simulink model "FogRectificationHDL"  (R2024b)
settings: Solver=FixedStepDiscrete  StartTime=0.0  StopTime=2*T  RelTol=1e-3
InitFcn:
  | img_path = get_param('FogRectificationHDL/FogImage','FileName');
  | img = imread(img_path);
  | %[m,n,c] = size(img);
  | m = 240;
  | n = 320;
  | c = 3;
  | dimI = [m n 3];
  | g = m*n;
  | 
  | numPixels = prod(dimI);
  | h1 = [1, 2, 1; 2, 4, 2; 1, 2 ,1]./16 ;
  | h = fliplr(flipud(h1));
  | T =324*402; % total pixels per line*total video lines
  | 
  | numBins = 256;
  | hazeFactor = 0.9;
  | reductionFactor = 0.6;
  | normFactor =  1/g;
  | threshold1 = 0.05;
  | threshold2 = 0.95;
  | o1 = 25;
  | o2 = 229;
  | o2_1 = 204;
  | max_o2 = 26;
undefined symbols (not defined in the file or in its folder): gray, Rec, SDTV
libraries: simulink x40, hdlsllib x32, visionhdlutilities x2, visionhdlio x2, visionsources x1, visionhdlstatistics x1, visionhdlconversions x1, visionhdlfilter x1, visionzynq_privlib x1
(part 1 of 2)
settings Model: DataTypeOverride=Off  ModifiedByFormat=The MathWorks, Inc.  SimulationMode=accelerator  Creator=The MathWorks, Inc.  LastModifiedBy=The MathWorks, Inc.
settings SolverCC: AlgebraicLoopSolver=TrustRegion
settings DataIOCC: SaveOutput=off  SaveTime=off
settings OptimizationCC: BlockReduction=off  ConditionallyExecuteInputs=off  DefaultParameterBehavior=Inlined
settings DebuggingCC: AlgebraicLoopMsg=error  SingleTaskRateTransMsg=error  ParameterPrecisionLossMsg=none  UnconnectedInputMsg=warning  UnconnectedOutputMsg=warning  UnconnectedLineMsg=warning
settings HardwareCC: ProdBitPerPointer=32  ProdBitPerSizeT=32  ProdBitPerPtrDiffT=32  ProdLargestAtomicFloat=None  ProdIntDivRoundTo=Undefined  ProdEndianess=Unspecified  ProdWordSize=32  ProdHWDeviceType=ASIC/FPGA->ASIC/FPGA  TargetBitPerLong=64  TargetBitPerPointer=64  TargetBitPerSizeT=64  TargetBitPerPtrDiffT=64  TargetLongLongMode=on  TargetIntDivRoundTo=Zero  TargetEndianess=LittleEndian  TargetWordSize=64  TargetHWDeviceType=Custom Processor->MATLAB Host Computer  ProdEqTarget=off
settings ModelReferenceCC: EnableRefExpFcnMdlSchedulingChecks=on
settings RTWCC: GPUComputeCapability=3.5  DLArmComputeVersion=19.05

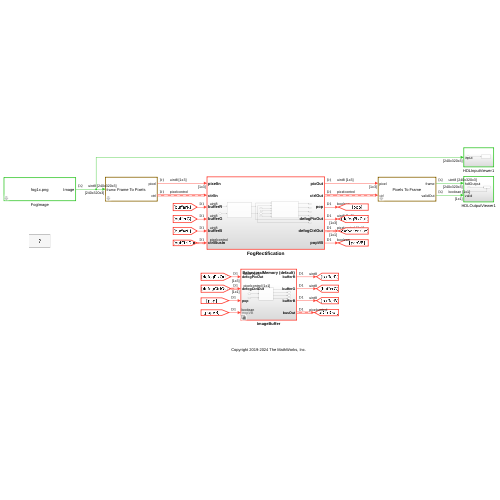
[thumbnail: Simulink's stored preview of the top-level diagram]
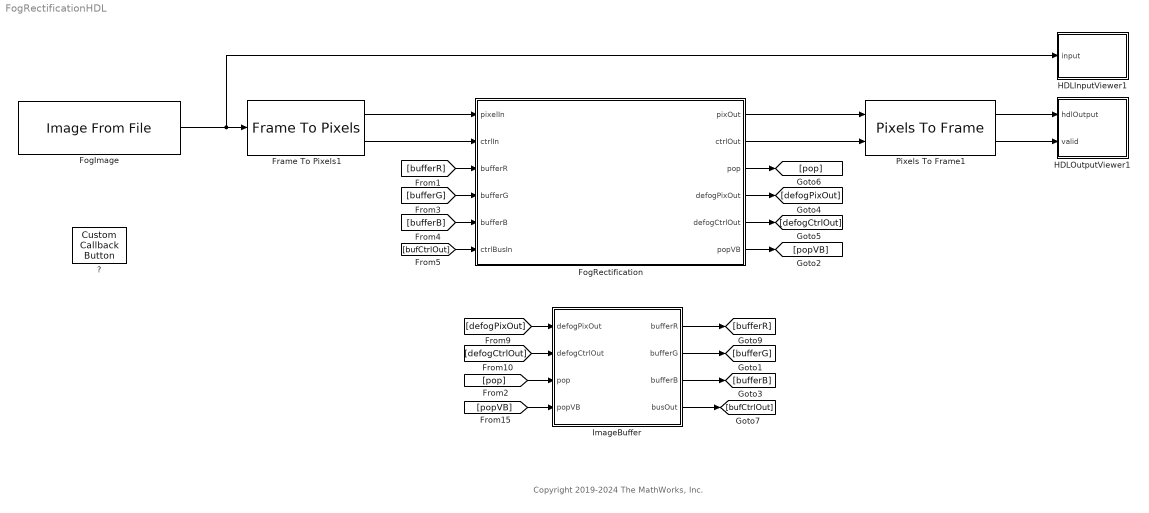
== system FogRectificationHDL ==
  note: Copyright 2019-2024 The MathWorks, Inc.
  "?" : CustomCallbackButton  Configuration="{\"components\":[{\"name\":\"BackgroundImageComponent\",\"settings\":{\"image\":{\"size\":[0,0],\"src\":\"default\",\"srcOrientation\":\"Right\"},\"position\":[0,0,1,1]}},{\"name\":\"ButtonStateComponent\",\"settings\":{\"buttonType\":\"momentary\",\"clickFcn\":\"showExample('visionhdl\\/FogRectificationHDLExample')\",\"onValue\":1,\"position\":[0,0,1,1],\"pressDelay\":\"500\",\"pressFcn\":\"\",\"repeatInterval\":\"0\",\"states\":[{\"horizontalAlignment\":\"center\",\"image\":{\"position\":[0,0,1,1],\"size\":[1,1],\"src\":\"default\",\"srcOrientation\":\"Right\"},\"label\":{\"color\":[0.01176470588,0.01176470588,0.01176470588,1],\"icon\":{\"size\":[0,0],\"src\":\"default\",\"srcOrientation\":\"Right\"},\"iconPlacement\":\"left\",\"opacity\":1,\"show\":true,\"text\":{\"content\":\"?\",\"font\":\"Helvetica\"}},\"labelOffset\":[0,0],\"verticalAlignment\":\"middle\"},{\"horizontalAlignment\":\"center\",\"image\":{\"position\":[0,0,1,1],\"size\":[1,1],\"src\":\"default\",\"srcOrientation\":\"Right\"},\"label\":{\"color\":[0.01176470588,0.01176470588,0.01176470588,1],\"icon\":{\"size\":[0,0],\"src\":\"default\",\"srcOrientation\":\"Right\"},\"iconPlacement\":\"left\",\"opacity\":1,\"show\":true,\"text\":{\"content\":\"?\",\"font\":\"Helvetica\"}},\"labelOffset\":[0,0],\"verticalAlignment\":\"middle\"},{\"horizontalAlignment\":\"center\",\"image\":{\"position\":[0,0,1,1],\"size\":[1,1],\"src\":\"default\",\"srcOrientation\":\"Right\"},\"label\":{\"color\":[0.01176470588,0.01176470588,0.01176470588,1],\"icon\":{\"size\":[0,0],\"src\":\"default\",\"srcOrientation\":\"Right\"},\"iconPlacement\":\"left\",\"opacity\":1,\"show\":true,\"text\":{\"content\":\"?\",\"font\":\"Helvetica\"}},\"labelOffset\":[0,0],\"verticalAlignment\":\"middle\"},{\"horizontalAlignment\":\"center\",\"image\":{\"position\":[0,0,1,1],\"size\":[1,1],\"src\":\"default\",\"srcOrientation\":\"Right\"},\"label\":{\"color\":[0.01176470588,0.01176470588,0.01176470588,1],\"icon\":{\"size\":[0,0],\"src\":\"default\",\"srcOrientation\":\"Right\"},\"iconPlacement\":\"left\",\"opacity\":1,\"show\":true,\"text\":{\"content\":\"?\",\"font\":\"Helvetica\"}},\"labelOffset\":[0,0],\"verticalAlignment\":\"middle\"}]}},{\"name\":\"ForegroundImageComponent\",\"settings\":{\"image\":{\"size\":[0,0],\"src\":\"default\",\"srcOrientation\":\"Right\"},\"isForeground\":1,\"position\":[0,0,1,1]}}],\"settings\":{\"BindingType\":\"standalone\",\"backgroundColor\":[244,244,244,1],\"backgroundOffset\":0,\"backgroundOpacity\":1,\"fixedAspectRatio\":\"off\",\"foregroundColor\":[0.01176470588,0.01176470588,0.01176470588,1],\"migratedFromLegacy\":true,\"useBackgroundColor\":true,\"variant\":\"callback\",\"version\":\"R2024b\"},\"type\":\"Button\"}"  CustomBackgroundColor="{\"color\":[0.9568627451,0.9568627451,0.9568627451],\"show\":true}"
  FogImage : visionsources/Image From File  Tag=vipblks_nd  FileName=./fog1x.png  Ts=T  imagePorts=One multidimensional signal  OutPortLabels=R|G|B  ImageDataType=Inherit from input image  sdImageDataType=uint(8)  Signed=on  WordLength=16  FractionLengthMode=User-defined  FractionLength=15
  FogRectification : Subsystem
  Frame To Pixels1 : visionhdlio/Frame To Pixels  NumComponents=3  NumPixels=1  VideoFormat=240p  ActivePixelsPerLine=320  ActiveVideoLines=240  TotalPixelsPerLine=402  TotalVideoLines=324  StartingActiveLine=1  FrontPorch=44  SampleTime=0  VideoFormatCache=240p  ActivePixelsPerLineCache=160  ActiveVideoLinesCache=160  TotalPixelsPerLineCache=400  TotalVideoLinesCache=400  StartingActiveLineCache=6  FrontPorchCache=120
  HDLInputViewer1 : Subsystem
  HDLOutputViewer1 : Subsystem
  ImageBuffer : Subsystem  Variant=on  VariantControlMode=label  LabelModeActiveChoice=(default)
  Pixels To Frame1 : visionhdlio/Pixels To Frame  NumComponents=3  NumPixels=1  VideoFormat=240p  ActivePixelsPerLine=320  ActiveVideoLines=240  TotalPixelsPerLine=402  TotalVideoLines=324  VideoFormatCache=240p  ActivePixelsPerLineCache=320  ActiveVideoLinesCache=240  TotalPixelsPerLineCache=402  TotalVideoLinesCache=324
  wires:
  FogRectification/6(popVB) -> [popVB]
  FogRectification/1(pixOut) -> Pixels To Frame1/1
  FogImage/1 -> HDLInputViewer1/1(input), Frame To Pixels1/1
  Pixels To Frame1/2 -> HDLOutputViewer1/2(valid)
  FogRectification/3(pop) -> [pop]
  [bufferR] -> FogRectification/3(bufferR)
  FogRectification/2(ctrlOut) -> Pixels To Frame1/2
  Pixels To Frame1/1 -> HDLOutputViewer1/1(hdlOutput)
  ImageBuffer/3(bufferB) -> [bufferB]
  [pop] -> ImageBuffer/3(pop)
  Frame To Pixels1/1 -> FogRectification/1(pixelIn)
  ImageBuffer/2(bufferG) -> [bufferG]
  Frame To Pixels1/2 -> FogRectification/2(ctrlIn)
  [bufferB] -> FogRectification/5(bufferB)
  FogRectification/5(defogCtrlOut) -> [defogCtrlOut]
  [defogPixOut] -> ImageBuffer/1(defogPixOut)
  FogRectification/4(defogPixOut) -> [defogPixOut]
  ImageBuffer/4(busOut) -> [bufCtrlOut]
  [popVB] -> ImageBuffer/4(popVB)
  ImageBuffer/1(bufferR) -> [bufferR]
  [defogCtrlOut] -> ImageBuffer/2(defogCtrlOut)
  [bufCtrlOut] -> FogRectification/6(ctrlBusIn)
  [bufferG] -> FogRectification/4(bufferG)

== system FogRectificationHDL/FogRectification ==
  pixelIn : Inport
  ctrlIn : Inport  Port=2
  bufferR : Inport  Port=3
  bufferG : Inport  Port=4
  bufferB : Inport  Port=5
  ctrlBusIn : Inport  Port=6
  ContrastEnhancement : Subsystem
  FogRemoval : Subsystem
  pixOut : Outport  VectorParamsAs1DForOutWhenUnconnected=off
  ctrlOut : Outport  Port=2  VectorParamsAs1DForOutWhenUnconnected=off
  pop : Outport  Port=3  VectorParamsAs1DForOutWhenUnconnected=off
  defogPixOut : Outport  Port=4  VectorParamsAs1DForOutWhenUnconnected=off
  defogCtrlOut : Outport  Port=5  VectorParamsAs1DForOutWhenUnconnected=off
  popVB : Outport  Port=6  VectorParamsAs1DForOutWhenUnconnected=off
  wires:
  pixelIn/1 -> FogRemoval/1(pixelIn)
  ctrlIn/1 -> FogRemoval/2(ctrlIn)
  FogRemoval/1(defogPixOut) -> ContrastEnhancement/1(pixelIn), defogPixOut/1
  FogRemoval/2(defogCtrlOut) -> ContrastEnhancement/2(ctrlIn), defogCtrlOut/1
  bufferR/1 -> ContrastEnhancement/3(bufferR)
  bufferG/1 -> ContrastEnhancement/4(bufferG)
  bufferB/1 -> ContrastEnhancement/5(bufferB)
  ContrastEnhancement/1(pixelOut) -> pixOut/1
  ContrastEnhancement/2(ctrlBusOut) -> ctrlOut/1
  ContrastEnhancement/3(pop) -> pop/1
  ctrlBusIn/1 -> ContrastEnhancement/6(ctrlBusIn)
  ContrastEnhancement/4(popVB) -> popVB/1

== system FogRectificationHDL/HDLInputViewer1 ==
  input : Inport
  hdlFogInput : VideoViewer  colormapValue=gray(256)  FigPos=[1217 942 673 613]
  wires:
  input/1 -> hdlFogInput/1

== system FogRectificationHDL/HDLOutputViewer1 ==
  hdlOutput : Inport
  valid : Inport  Port=2
  HDLOutputViewer : Subsystem
  wires:
  hdlOutput/1 -> HDLOutputViewer/1(h)
  valid/1 -> HDLOutputViewer/Enable

== system FogRectificationHDL/ImageBuffer ==
  note: 1) Add Subsystem or Model blocks as valid variant choices.
      | 2) You cannot connect blocks at this level. At simulation, connectivity is automatically
      | determined, based on the active variant and port name matching.
  note: 1) Behavioral Memory and VideoFrameBuffer are the two variant choices.
      | 2) Behavioral Memory is designed using HDL FIFO blocks.
      | 3) VideoFrameBuffer block is used from xilinxzynqbasedvision supportPkg.
      | 4) Currently VideoFrameBuffer block is used only for Simulation.
      | 5) For FPGA-in-the-Loop Simulations, make sure Behavioral Memory is enabled.
  defogPixOut : Inport
  defogCtrlOut : Inport  Port=2
  pop : Inport  Port=3
  popVB : Inport  Port=4
  BehavioralMemory : Subsystem  VariantControl=(default)
  VideoFrameBuffer : Subsystem  VariantControl=VideoFrameBuffer
  bufferR : Outport
  bufferG : Outport  Port=2
  bufferB : Outport  Port=3
  busOut : Outport  Port=4

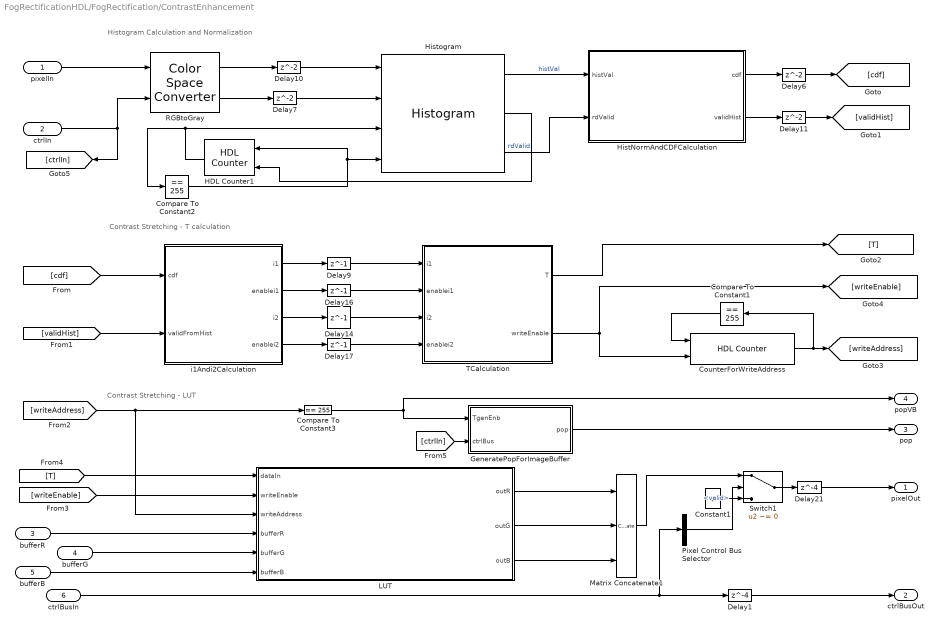
== system FogRectificationHDL/FogRectification/ContrastEnhancement ==
  note: Histogram Calculation and Normalization
  note: Contrast Stretching - LUT
  note: Contrast Stretching - T calculation
  pixelIn : Inport
  ctrlIn : Inport  Port=2
  bufferR : Inport  Port=3
  bufferG : Inport  Port=4
  bufferB : Inport  Port=5
  ctrlBusIn : Inport  Port=6
  Compare To Constant1 : simulink/Logic and Bit Operations/Compare To Constant  relop===  const=255  OutDataTypeStr=boolean
  Compare To Constant2 : simulink/Logic and Bit Operations/Compare To Constant  relop===  const=255  OutDataTypeStr=boolean
  Compare To Constant3 : simulink/Logic and Bit Operations/Compare To Constant  relop===  const=255  OutDataTypeStr=boolean
  Constant1 : Constant  Value=0  OutDataTypeStr=uint8  SampleTime=-1
  CounterForWriteAddress : hdlsllib/Sources/HDL Counter  CountType=Free running  CountInit=0  CountStep=1  CountMax=25  CountFromType=Initial value  CountFrom=0  CountResetPort=on  CountLoadPort=off  CountEnbPort=on  CountDirPort=off  CountHitOutputPort=off  CountDataType=Unsigned  CountWordLen=8  CountFracLen=0  CountSampTime=1
  Delay1 : Delay  DelayLength=4
  Delay{6..7,10..11} (4 alike) : Delay
  Delay{9,14,16..17} (4 alike) : Delay  DelayLength=1
  Delay21 : Delay  DelayLength=4
  GeneratePopForImageBuffer : Subsystem
  HDL Counter1 : hdlsllib/Sources/HDL Counter  CountType=Count limited  CountInit=0  CountStep=1  CountMax=255  CountFromType=Initial value  CountFrom=0  CountResetPort=on  CountLoadPort=off  CountEnbPort=on  CountDirPort=off  CountHitOutputPort=off  CountDataType=Unsigned  CountWordLen=ceil(log2(numBins))  CountFracLen=0  CountSampTime=1
  HistNormAndCDFCalculation : Subsystem
  Histogram : visionhdlstatistics/Histogram  NumBins=256  OutputDataType=Unsigned fixed point  OutputWL=16  SimulateUsing=Code generation
  LUT : Subsystem
  Matrix Concatenate1 : Concatenate  NumInputs=3  Mode=Multidimensional array  ConcatenateDimension=2
  Pixel Control Bus Selector : BusSelector  OutputSignals=valid
  RGBtoGray : visionhdlconversions/Color Space Converter  Conversion=RGB to intensity  ConversionStandard=Rec. 601 (SDTV)  ScanningStandard=1250/50/2:1  SimulateUsing=Code generation
  Switch1 : Switch  Criteria=u2 ~= 0  SaturateOnIntegerOverflow=off  InputSameDT=off
  TCalculation : Subsystem
  i1Andi2Calculation : Subsystem
  pixelOut : Outport
  ctrlBusOut : Outport  Port=2
  pop : Outport  Port=3
  popVB : Outport  Port=4
  wires:
  TCalculation/1(T) -> [T]
  CounterForWriteAddress/1 -> Compare To Constant1/1, [writeAddress]
  i1Andi2Calculation/4(enablei2) -> Delay17/1
  i1Andi2Calculation/3(i2) -> Delay14/1
  i1Andi2Calculation/1(i1) -> Delay9/1
  i1Andi2Calculation/2(enablei1) -> Delay16/1
  Delay17/1 -> TCalculation/4(enablei2)
  Delay14/1 -> TCalculation/3(i2)
  Delay9/1 -> TCalculation/1(i1)
  Delay16/1 -> TCalculation/2(enablei1)
  [cdf] -> i1Andi2Calculation/1(cdf)
  [validHist] -> i1Andi2Calculation/2(validFromHist)
  Delay6/1 -> [cdf]
  Delay11/1 -> [validHist]
  GeneratePopForImageBuffer/1(pop) -> pop/1
  Switch1/1 -> Delay21/1
  [writeAddress] -> LUT/3(writeAddress), Compare To Constant3/1
  LUT/1(outR) -> Matrix Concatenate1/1
  LUT/3(outB) -> Matrix Concatenate1/3
  bufferR/1 -> LUT/4(bufferR)
  bufferG/1 -> LUT/5(bufferG)
  [writeEnable] -> LUT/2(writeEnable)
  [T] -> LUT/1(dataIn)
  LUT/2(outG) -> Matrix Concatenate1/2
  bufferB/1 -> LUT/6(bufferB)
  Constant1/1 -> Switch1/3
  Compare To Constant3/1 -> GeneratePopForImageBuffer/1(TgenEnb), popVB/1
  Matrix Concatenate1/1 -> Switch1/1
  ctrlBusIn/1 -> Delay1/1, Pixel Control Bus Selector/1
  Delay21/1 -> pixelOut/1
  Pixel Control Bus Selector/1 -> Switch1/2  "<valid>"
  [ctrlIn] -> GeneratePopForImageBuffer/2(ctrlBus)
  Delay7/1 -> Histogram/2
  Delay10/1 -> Histogram/1
  HDL Counter1/1 -> Histogram/3, Compare To Constant2/1
  RGBtoGray/2 -> Delay7/1
  RGBtoGray/1 -> Delay10/1
  Compare To Constant2/1 -> HDL Counter1/1, Histogram/4
  Histogram/2 -> HDL Counter1/2
  pixelIn/1 -> RGBtoGray/1
  ctrlIn/1 -> RGBtoGray/2, [ctrlIn]
  Histogram/1 -> HistNormAndCDFCalculation/1(histVal)  "histVal"
  Histogram/3 -> HistNormAndCDFCalculation/2(rdValid)  "rdValid"
  HistNormAndCDFCalculation/1(cdf) -> Delay6/1
  HistNormAndCDFCalculation/2(validHist) -> Delay11/1
  TCalculation/2(writeEnable) -> CounterForWriteAddress/2, [writeEnable]
  Delay1/1 -> ctrlBusOut/1
  Compare To Constant1/1 -> CounterForWriteAddress/1

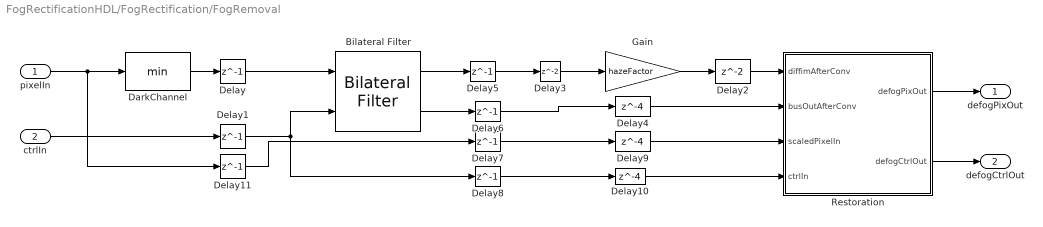
== system FogRectificationHDL/FogRectification/FogRemoval ==
  pixelIn : Inport
  ctrlIn : Inport  Port=2
  Bilateral Filter : visionhdlfilter/Bilateral Filter  NeighborhoodSize=3x3  SpatialStdDev=2  IntensityStdDev=0.5  PaddingMethod=Constant  PaddingValue=0  LineBufferSize=2048  SimulateUsing=Code generation  CoefficientsDataTypeStr=fixdt(0,11,10)  roundingMode=Floor  overflowMode=on  OutputMin=[]  OutputMax=[]
  DarkChannel : MinMax  OutDataTypeStr=uint8
  Delay{,1,5..8,11} (7 alike) : Delay  DelayLength=1
  Delay10 : Delay  DelayLength=4
  Delay2 : Delay
  Delay3 : Delay
  Delay4 : Delay  DelayLength=4
  Delay9 : Delay  DelayLength=4
  Gain : Gain  Gain=hazeFactor  ParamDataTypeStr=fixdt(0,16,15)
  Restoration : Subsystem
  defogPixOut : Outport
  defogCtrlOut : Outport  Port=2
  wires:
  DarkChannel/1 -> Delay/1
  ctrlIn/1 -> Delay1/1
  pixelIn/1 -> Delay11/1, DarkChannel/1
  Delay10/1 -> Restoration/4(ctrlIn)
  Restoration/1(defogPixOut) -> defogPixOut/1
  Delay11/1 -> Delay7/1
  Delay9/1 -> Restoration/3(scaledPixelIn)
  Restoration/2(defogCtrlOut) -> defogCtrlOut/1
  Delay2/1 -> Restoration/1(diffimAfterConv)
  Delay4/1 -> Restoration/2(busOutAfterConv)
  Delay7/1 -> Delay9/1
  Delay8/1 -> Delay10/1
  Delay6/1 -> Delay4/1
  Gain/1 -> Delay2/1
  Delay3/1 -> Gain/1
  Delay5/1 -> Delay3/1
  Bilateral Filter/2 -> Delay6/1
  Bilateral Filter/1 -> Delay5/1
  Delay1/1 -> Delay8/1, Bilateral Filter/2
  Delay/1 -> Bilateral Filter/1

== system FogRectificationHDL/HDLOutputViewer1/HDLOutputViewer ==
  h : Inport
  Enable : EnablePort
  hdlFogOutput : VideoViewer  colormapValue=gray(256)  FigPos=[48 912 1348 650]
  wires:
  h/1 -> hdlFogOutput/1

== system FogRectificationHDL/ImageBuffer/BehavioralMemory ==
  defogPixOut : Inport
  defogCtrlOut : Inport  Port=2
  pop : Inport  Port=3
  BehavioralMemory : Subsystem
  bufferR : Outport
  bufferG : Outport  Port=2
  bufferB : Outport  Port=3
  busOut : Outport  Port=4
  wires:
  defogPixOut/1 -> BehavioralMemory/1(defogPixOut)
  pop/1 -> BehavioralMemory/3(pop)
  defogCtrlOut/1 -> BehavioralMemory/2(defogCtrlOut)
  BehavioralMemory/1(bufferOpR) -> bufferR/1
  BehavioralMemory/2(buferOpG) -> bufferG/1
  BehavioralMemory/3(bufferOpB) -> bufferB/1
  BehavioralMemory/4(busOut) -> busOut/1

== system FogRectificationHDL/ImageBuffer/VideoFrameBuffer ==
  defogPixOut : Inport
  defogCtrlOut : Inport  Port=2
  popVB : Inport  Port=3
  Delay : Delay  DelayLength=1
  Demux : Demux  Outputs=3
  Video Frame Buffer : visionzynq_privlib/Video Frame Buffer  FrameSize=320x240p  ColorSpace=RGB  mask(Frame Buffer Simulation){}
  bufferR : Outport
  bufferG : Outport  Port=2
  bufferB : Outport  Port=3
  busOut : Outport  Port=4
  wires:
  Video Frame Buffer/2 -> bufferG/1
  Video Frame Buffer/1 -> bufferR/1
  Video Frame Buffer/4 -> Delay/1
  popVB/1 -> Video Frame Buffer/5
  defogCtrlOut/1 -> Video Frame Buffer/4
  defogPixOut/1 -> Demux/1
  Demux/1 -> Video Frame Buffer/1
  Demux/2 -> Video Frame Buffer/2
  Demux/3 -> Video Frame Buffer/3
  Video Frame Buffer/3 -> bufferB/1
  Delay/1 -> busOut/1

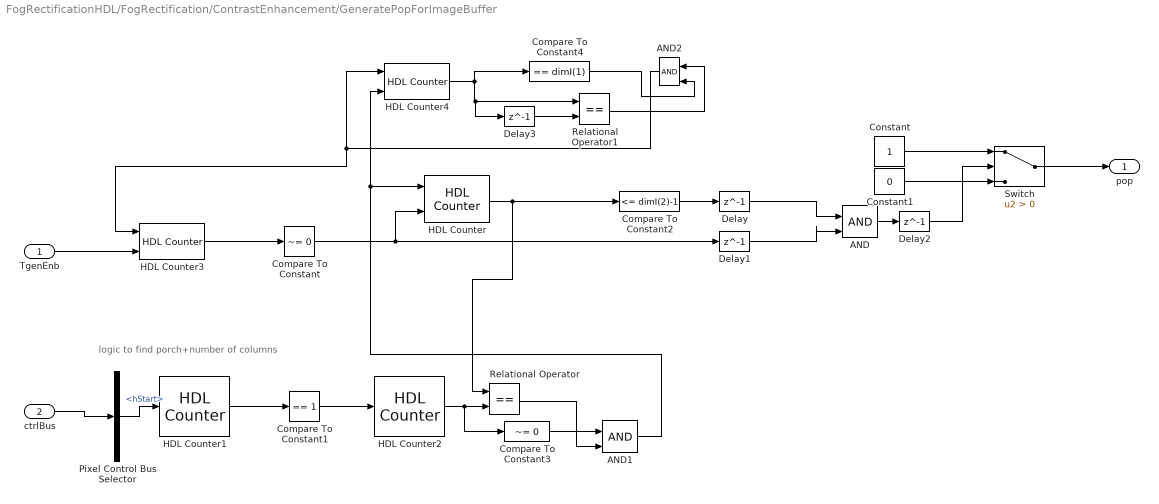
== system FogRectificationHDL/FogRectification/ContrastEnhancement/GeneratePopForImageBuffer ==
  note: logic to find porch+number of columns
  TgenEnb : Inport
  ctrlBus : Inport  Port=2
  AND : Logic  IconShape=distinctive  AllPortsSameDT=off  OutDataTypeStr=boolean
  AND1 : Logic  IconShape=distinctive  AllPortsSameDT=off  OutDataTypeStr=boolean
  AND2 : Logic  IconShape=distinctive  AllPortsSameDT=off  OutDataTypeStr=boolean
  Compare To Constant : simulink/Logic and Bit Operations/Compare To Constant  relop=~=  const=0  OutDataTypeStr=boolean
  Compare To Constant1 : simulink/Logic and Bit Operations/Compare To Constant  relop===  const=1  OutDataTypeStr=boolean
  Compare To Constant2 : simulink/Logic and Bit Operations/Compare To Constant  relop=<=  const=dimI(2)-1  OutDataTypeStr=boolean
  Compare To Constant3 : simulink/Logic and Bit Operations/Compare To Constant  relop=~=  const=0  OutDataTypeStr=boolean
  Compare To Constant4 : simulink/Logic and Bit Operations/Compare To Constant  relop===  const=dimI(1)  OutDataTypeStr=boolean
  Constant : Constant  OutDataTypeStr=boolean  SampleTime=-1
  Constant1 : Constant  Value=0  OutDataTypeStr=boolean  SampleTime=-1
  Delay{,1..3} (4 alike) : Delay  DelayLength=1
  HDL Counter : hdlsllib/Sources/HDL Counter  CountType=Free running  CountInit=0  CountStep=1  CountMax=399  CountFromType=Initial value  CountFrom=0  CountResetPort=on  CountLoadPort=off  CountEnbPort=on  CountDirPort=off  CountHitOutputPort=off  CountDataType=Unsigned  CountWordLen=17  CountFracLen=0  CountSampTime=1
  HDL Counter1 : hdlsllib/Sources/HDL Counter  CountType=Free running  CountInit=0  CountStep=1  CountMax=25  CountFromType=Initial value  CountFrom=0  CountResetPort=off  CountLoadPort=off  CountEnbPort=on  CountDirPort=off  CountHitOutputPort=off  CountDataType=Unsigned  CountWordLen=16  CountFracLen=0  CountSampTime=1
  HDL Counter2 : hdlsllib/Sources/HDL Counter  CountType=Free running  CountInit=0  CountStep=1  CountMax=25  CountFromType=Initial value  CountFrom=0  CountResetPort=off  CountLoadPort=off  CountEnbPort=on  CountDirPort=off  CountHitOutputPort=off  CountDataType=Unsigned  CountWordLen=16  CountFracLen=0  CountSampTime=1
  HDL Counter3 : hdlsllib/Sources/HDL Counter  CountType=Free running  CountInit=0  CountStep=1  CountMax=399  CountFromType=Initial value  CountFrom=0  CountResetPort=on  CountLoadPort=off  CountEnbPort=on  CountDirPort=off  CountHitOutputPort=off  CountDataType=Unsigned  CountWordLen=17  CountFracLen=0  CountSampTime=1
  HDL Counter4 : hdlsllib/Sources/HDL Counter  CountType=Free running  CountInit=0  CountStep=1  CountMax=25  CountFromType=Initial value  CountFrom=0  CountResetPort=on  CountLoadPort=off  CountEnbPort=on  CountDirPort=off  CountHitOutputPort=off  CountDataType=Unsigned  CountWordLen=16  CountFracLen=0  CountSampTime=1
  Pixel Control Bus Selector : BusSelector  OutputSignals=hStart
  Relational Operator : RelationalOperator  Operator===  OutDataTypeStr=boolean  RndMeth=Simplest  InputSameDT=off
  Relational Operator1 : RelationalOperator  Operator===  OutDataTypeStr=boolean  RndMeth=Simplest  InputSameDT=off
  Switch : Switch  Criteria=u2 > Threshold  OutDataTypeStr=boolean  SaturateOnIntegerOverflow=off  InputSameDT=off
  pop : Outport
  wires:
  Constant/1 -> Switch/1
  Constant1/1 -> Switch/3
  Switch/1 -> pop/1
  AND/1 -> Delay2/1
  Compare To Constant2/1 -> Delay/1
  HDL Counter3/1 -> Compare To Constant/1
  Delay1/1 -> AND/2
  Delay2/1 -> Switch/2
  Relational Operator/1 -> AND1/2
  ctrlBus/1 -> Pixel Control Bus Selector/1
  HDL Counter/1 -> Compare To Constant2/1, Relational Operator/1
  Pixel Control Bus Selector/1 -> HDL Counter1/1  "<hStart>"
  Compare To Constant3/1 -> AND1/1
  HDL Counter4/1 -> Relational Operator1/1, Delay3/1, Compare To Constant4/1
  Delay3/1 -> Relational Operator1/2
  Relational Operator1/1 -> AND2/1
  Compare To Constant4/1 -> AND2/2
  Delay/1 -> AND/1
  AND2/1 -> HDL Counter3/1, HDL Counter4/1
  AND1/1 -> HDL Counter/1, HDL Counter4/2
  Compare To Constant/1 -> Delay1/1, HDL Counter/2
  TgenEnb/1 -> HDL Counter3/2
  Compare To Constant1/1 -> HDL Counter2/1
  HDL Counter1/1 -> Compare To Constant1/1
  HDL Counter2/1 -> Compare To Constant3/1, Relational Operator/2

== system FogRectificationHDL/FogRectification/ContrastEnhancement/HistNormAndCDFCalculation ==
  histVal : Inport
  rdValid : Inport  Port=2
  Add : Sum
  Constant : Constant  Value=0  OutDataTypeStr=Inherit: Inherit via back propagation  SampleTime=-1
  Data Type Conversion : DataTypeConversion  OutDataTypeStr=fixdt(0,32,16)  RndMeth=Nearest  SaturateOnIntegerOverflow=off
  Delay{2..5} (4 alike) : Delay
  Delay20 : Delay  DelayLength=1
  Delay8 : Delay  DelayLength=1
  Gain : Gain  Gain=normFactor  ParamDataTypeStr=fixdt(0,16,31)  OutDataTypeStr=fixdt(0,32,16)  RndMeth=Nearest
  Switch : Switch  Criteria=u2 > Threshold  SaturateOnIntegerOverflow=off  InputSameDT=off
  cdf : Outport
  validHist : Outport  Port=2
  wires:
  Delay8/1 -> validHist/1, Switch/2
  Delay3/1 -> Delay5/1
  Delay2/1 -> Data Type Conversion/1
  Delay5/1 -> Delay8/1
  Switch/1 -> cdf/1, Add/1
  histVal/1 -> Delay2/1
  Delay20/1 -> Switch/1
  Gain/1 -> Delay4/1
  Data Type Conversion/1 -> Gain/1
  Constant/1 -> Switch/3
  Delay4/1 -> Add/2
  Add/1 -> Delay20/1
  rdValid/1 -> Delay3/1

== system FogRectificationHDL/FogRectification/ContrastEnhancement/LUT ==
  dataIn : Inport
  writeEnable : Inport  Port=2
  writeAddress : Inport  Port=3
  bufferR : Inport  Port=4
  bufferG : Inport  Port=5
  bufferB : Inport  Port=6
  InputBuffer : hdlsllib/HDL RAMs/Simple Dual Port RAM System  RAMType=Simple dual port  AsyncRead=off  WriteOutputValue=New data  RAMInitialValue=0  allowBusInputs=off  WritesHaveOutput=on  NumReads=0  NumWrites=1  SimulateUsing=Code generation  ModelRAMDelay=on
  InputBuffer1 : hdlsllib/HDL RAMs/Simple Dual Port RAM System  RAMType=Simple dual port  AsyncRead=off  WriteOutputValue=New data  RAMInitialValue=0  allowBusInputs=off  WritesHaveOutput=on  NumReads=0  NumWrites=1  SimulateUsing=Code generation  ModelRAMDelay=on
  InputBuffer2 : hdlsllib/HDL RAMs/Simple Dual Port RAM System  RAMType=Simple dual port  AsyncRead=off  WriteOutputValue=New data  RAMInitialValue=0  allowBusInputs=off  WritesHaveOutput=on  NumReads=0  NumWrites=1  SimulateUsing=Code generation  ModelRAMDelay=on
  outR : Outport
  outG : Outport  Port=2
  outB : Outport  Port=3
  wires:
  dataIn/1 -> InputBuffer2/1, InputBuffer1/1, InputBuffer/1
  InputBuffer1/1 -> outG/1
  writeEnable/1 -> InputBuffer2/3, InputBuffer1/3, InputBuffer/3
  writeAddress/1 -> InputBuffer/2, InputBuffer1/2, InputBuffer2/2
  InputBuffer/1 -> outR/1
  InputBuffer2/1 -> outB/1
  bufferR/1 -> InputBuffer/4
  bufferG/1 -> InputBuffer1/4
  bufferB/1 -> InputBuffer2/4

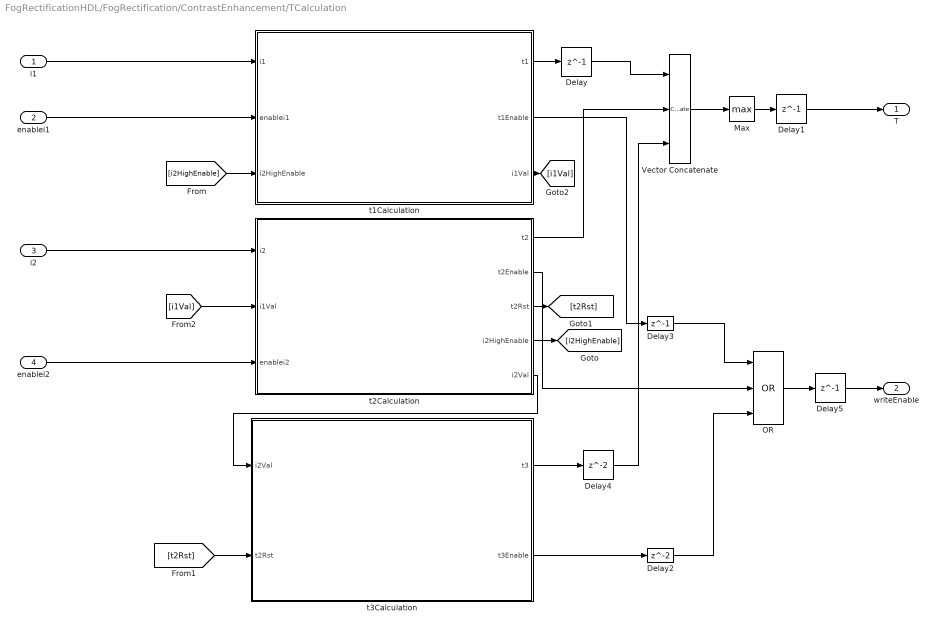
== system FogRectificationHDL/FogRectification/ContrastEnhancement/TCalculation ==
  i1 : Inport
  enablei1 : Inport  Port=2
  i2 : Inport  Port=3
  enablei2 : Inport  Port=4
  Delay{,1,3,5} (4 alike) : Delay  DelayLength=1
  Delay2 : Delay
  Delay4 : Delay
  Max : MinMax  Function=max
  OR : Logic  Operator=OR  Inputs=3  IconShape=distinctive  AllPortsSameDT=off  OutDataTypeStr=boolean
  Vector Concatenate : Concatenate  NumInputs=3
  t1Calculation : Subsystem
  t2Calculation : Subsystem
  t3Calculation : Subsystem
  T : Outport
  writeEnable : Outport  Port=2
  wires:
  i2/1 -> t2Calculation/1(i2)
  i1/1 -> t1Calculation/1(i1)
  enablei1/1 -> t1Calculation/2(enablei1)
  t1Calculation/1(t1) -> Delay/1
  enablei2/1 -> t2Calculation/3(enablei2)
  Vector Concatenate/1 -> Max/1
  Delay1/1 -> T/1
  Max/1 -> Delay1/1
  t2Calculation/2(t2Enable) -> OR/2
  OR/1 -> Delay5/1
  t2Calculation/4(i2HighEnable) -> [i2HighEnable]
  [i2HighEnable] -> t1Calculation/3(i2HighEnable)
  t2Calculation/3(t2Rst) -> [t2Rst]
  [t2Rst] -> t3Calculation/2(t2Rst)
  Delay/1 -> Vector Concatenate/1
  t2Calculation/1(t2) -> Vector Concatenate/2
  t3Calculation/1(t3) -> Delay4/1
  t3Calculation/2(t3Enable) -> Delay2/1
  t1Calculation/2(t1Enable) -> Delay3/1
  Delay2/1 -> OR/3
  Delay3/1 -> OR/1
  t2Calculation/5(i2Val) -> t3Calculation/1(i2Val)
  t1Calculation/3(i1Val) -> [i1Val]
  [i1Val] -> t2Calculation/2(i1Val)
  Delay4/1 -> Vector Concatenate/3
  Delay5/1 -> writeEnable/1

== system FogRectificationHDL/FogRectification/ContrastEnhancement/i1Andi2Calculation ==
  cdf : Inport
  validFromHist : Inport  Port=2
  "i1Calculation  " : Subsystem
  i2Calculation : Subsystem
  i1 : Outport
  enablei1 : Outport  Port=2
  i2 : Outport  Port=3
  enablei2 : Outport  Port=4
  wires:
  cdf/1 -> i2Calculation/1(cdf), "i1Calculation  "/1(cdf)
  "i1Calculation  "/2(enablei1) -> enablei1/1
  validFromHist/1 -> i2Calculation/2(validFromHist), "i1Calculation  "/2(validFromHist)
  "i1Calculation  "/1(i1) -> i1/1
  i2Calculation/1(i2) -> i2/1
  i2Calculation/2(enablei2) -> enablei2/1

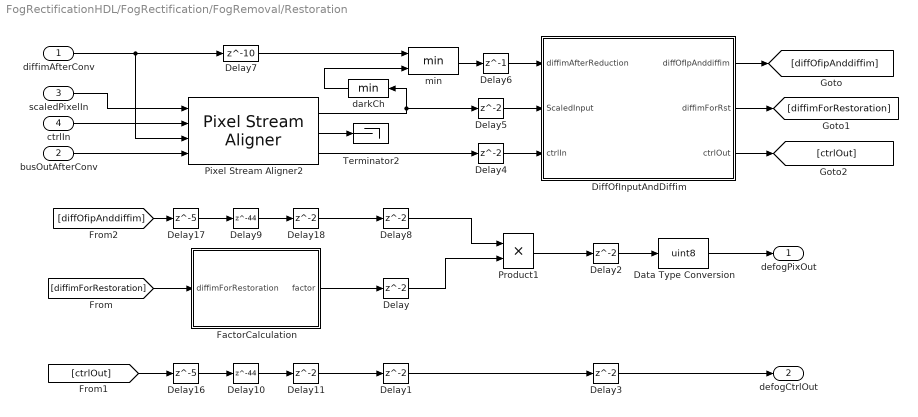
== system FogRectificationHDL/FogRectification/FogRemoval/Restoration ==
  diffimAfterConv : Inport
  busOutAfterConv : Inport  Port=2
  scaledPixelIn : Inport  Port=3
  ctrlIn : Inport  Port=4
  Data Type Conversion : DataTypeConversion  OutDataTypeStr=uint8  RndMeth=Nearest  SaturateOnIntegerOverflow=off
  Delay{,1..5,8,11,18} (9 alike) : Delay
  Delay10 : Delay  DelayLength=44
  Delay16 : Delay  DelayLength=5
  Delay17 : Delay  DelayLength=5
  Delay6 : Delay  DelayLength=1
  Delay7 : Delay  DelayLength=10
  Delay9 : Delay  DelayLength=44
  DiffOfInputAndDiffim : Subsystem
  FactorCalculation : Subsystem
  Pixel Stream Aligner2 : visionhdlutilities/Pixel Stream Aligner  LineBufferSize=n  MaximumNumberOfLines=15  SimulateUsing=Code generation
  Product1 : Product  OutDataTypeStr=fixdt(0,32,20)  RndMeth=Nearest
  Terminator2 : Terminator
  darkCh : MinMax  OutDataTypeStr=uint8
  min : MinMax  Inputs=2
  defogPixOut : Outport  VectorParamsAs1DForOutWhenUnconnected=off
  defogCtrlOut : Outport  Port=2  VectorParamsAs1DForOutWhenUnconnected=off
  wires:
  scaledPixelIn/1 -> Pixel Stream Aligner2/1
  min/1 -> Delay6/1
  Pixel Stream Aligner2/3 -> Delay4/1
  ctrlIn/1 -> Pixel Stream Aligner2/2
  Pixel Stream Aligner2/2 -> Terminator2/1
  diffimAfterConv/1 -> Delay7/1, Pixel Stream Aligner2/3
  busOutAfterConv/1 -> Pixel Stream Aligner2/4
  Delay2/1 -> Data Type Conversion/1
  Delay/1 -> Product1/2
  Product1/1 -> Delay2/1
  Delay11/1 -> Delay1/1
  Pixel Stream Aligner2/1 -> darkCh/1, Delay5/1
  darkCh/1 -> min/2
  Delay7/1 -> min/1
  Delay6/1 -> DiffOfInputAndDiffim/1(diffimAfterReduction)
  Delay5/1 -> DiffOfInputAndDiffim/2(ScaledInput)
  Delay4/1 -> DiffOfInputAndDiffim/3(ctrlIn)
  DiffOfInputAndDiffim/3(ctrlOut) -> [ctrlOut]
  DiffOfInputAndDiffim/2(diffimForRst) -> [diffimForRestoration]
  DiffOfInputAndDiffim/1(diffOfIpAnddiffim) -> [diffOfipAnddiffim]
  Delay3/1 -> defogCtrlOut/1
  Data Type Conversion/1 -> defogPixOut/1
  Delay8/1 -> Product1/1
  Delay1/1 -> Delay3/1
  [diffOfipAnddiffim] -> Delay17/1
  Delay18/1 -> Delay8/1
  [ctrlOut] -> Delay16/1
  Delay16/1 -> Delay10/1
  [diffimForRestoration] -> FactorCalculation/1(diffimForRestoration)
  FactorCalculation/1(factor) -> Delay/1
  Delay17/1 -> Delay9/1
  Delay9/1 -> Delay18/1
  Delay10/1 -> Delay11/1

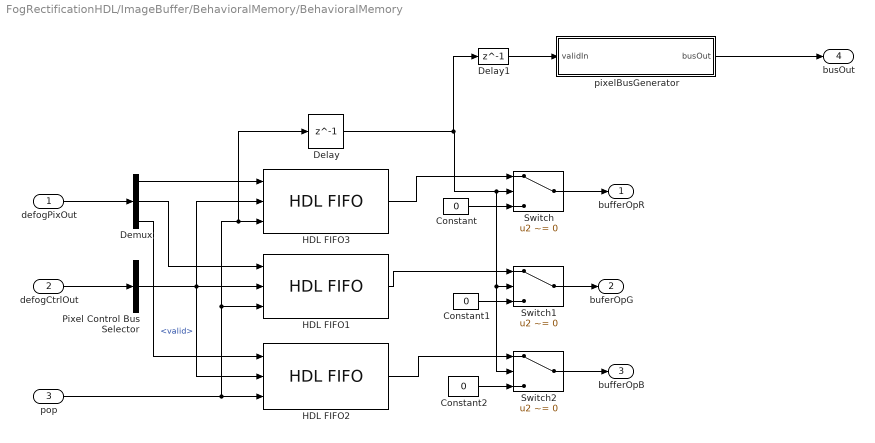
== system FogRectificationHDL/ImageBuffer/BehavioralMemory/BehavioralMemory ==
  defogPixOut : Inport
  defogCtrlOut : Inport  Port=2
  pop : Inport  Port=3
  Constant : Constant  Value=0  SampleTime=-1
  Constant1 : Constant  Value=0  SampleTime=-1
  Constant2 : Constant  Value=0  SampleTime=-1
  Delay : Delay  DelayLength=1
  Delay1 : Delay  DelayLength=1
  Demux : Demux  Outputs=3
  HDL FIFO1 : hdlsllib/HDL RAMs/HDL FIFO  fifo_size=g  mode=Classic  ratio=1  push_msg=Warning  pop_msg=Warning  show_empty=off  show_full=off  show_num=off  LabelModeActiveChoice_Mode=Classic  rst_port=off
  HDL FIFO2 : hdlsllib/HDL RAMs/HDL FIFO  fifo_size=g  mode=Classic  ratio=1  push_msg=Warning  pop_msg=Warning  show_empty=off  show_full=off  show_num=off  LabelModeActiveChoice_Mode=Classic  rst_port=off
  HDL FIFO3 : hdlsllib/HDL RAMs/HDL FIFO  fifo_size=g  mode=Classic  ratio=1  push_msg=Warning  pop_msg=Warning  show_empty=off  show_full=off  show_num=off  LabelModeActiveChoice_Mode=Classic  rst_port=off
  Pixel Control Bus Selector : BusSelector  OutputSignals=valid
  Switch : Switch  Criteria=u2 ~= 0  OutDataTypeStr=uint8  SaturateOnIntegerOverflow=off  InputSameDT=off
  Switch1 : Switch  Criteria=u2 ~= 0  OutDataTypeStr=uint8  SaturateOnIntegerOverflow=off  InputSameDT=off
  Switch2 : Switch  Criteria=u2 ~= 0  OutDataTypeStr=uint8  SaturateOnIntegerOverflow=off  InputSameDT=off
  pixelBusGenerator : Subsystem  mask{hEnd=dimI(2)-1, vEnd=dimI(1)*dimI(2) - 1}
      mask prompts: hEnd "hEnd Count"; vEnd "vEnd Count"
      mask DialogControl DescGroupVar Prompt: Counter Values
  bufferOpR : Outport
  buferOpG : Outport  Port=2
  bufferOpB : Outport  Port=3
  busOut : Outport  Port=4
  wires:
  Pixel Control Bus Selector/1 -> HDL FIFO3/2, HDL FIFO2/2, HDL FIFO1/2  "<valid>"
  Demux/2 -> HDL FIFO1/1
  Demux/3 -> HDL FIFO2/1
  Demux/1 -> HDL FIFO3/1
  defogPixOut/1 -> Demux/1
  defogCtrlOut/1 -> Pixel Control Bus Selector/1
  pop/1 -> Delay/1, HDL FIFO3/3, HDL FIFO1/3, HDL FIFO2/3
  Constant/1 -> Switch/3
  Switch/1 -> bufferOpR/1
  HDL FIFO1/1 -> Switch1/1
  Constant1/1 -> Switch1/3
  Switch1/1 -> buferOpG/1
  Switch2/1 -> bufferOpB/1
  Constant2/1 -> Switch2/3
  HDL FIFO2/1 -> Switch2/1
  Delay/1 -> Delay1/1, Switch2/2, Switch1/2, Switch/2
  pixelBusGenerator/1(busOut) -> busOut/1
  Delay1/1 -> pixelBusGenerator/1(validIn)
  HDL FIFO3/1 -> Switch/1

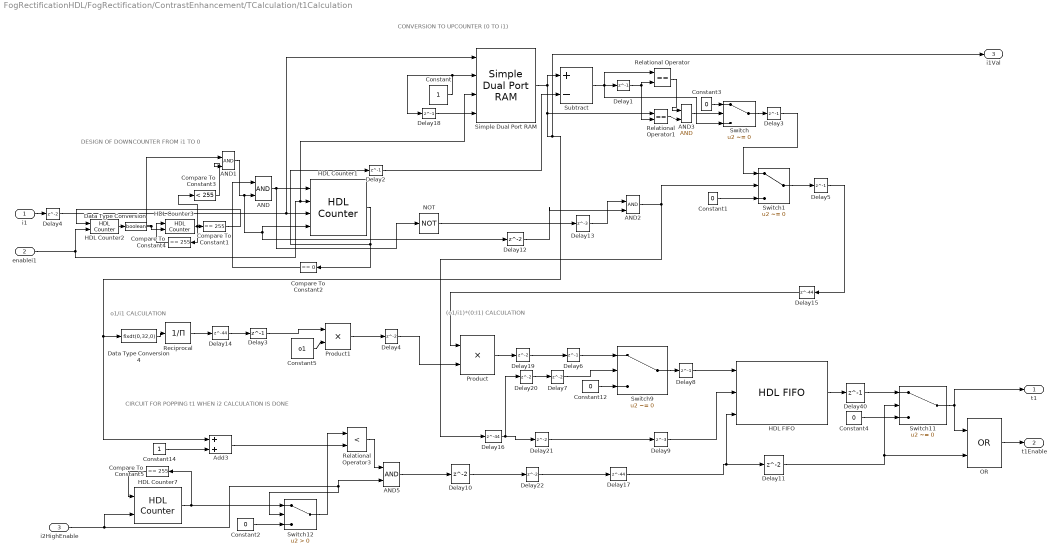
== system FogRectificationHDL/FogRectification/ContrastEnhancement/TCalculation/t1Calculation ==
  note: (o1/i1)*(0:I1) CALCULATION
  note: o1/i1 CALCULATION
  note: CONVERSION TO UPCOUNTER (0 TO i1)
  note: DESIGN OF DOWNCOUNTER FROM i1 TO 0
  note: CIRCUIT FOR POPPING t1 WHEN i2 CALCULATION IS DONE
  i1 : Inport
  enablei1 : Inport  Port=2
  i2HighEnable : Inport  Port=3
  " Delay3" : Delay  DelayLength=1
  " Delay4" : Delay
  AND{,1..3,5} (5 alike) : Logic  IconShape=distinctive  AllPortsSameDT=off  OutDataTypeStr=boolean
  Add3 : Sum  OutDataTypeStr=uint8
  Compare To Constant1 : simulink/Logic and Bit Operations/Compare To Constant  relop===  const=255  OutDataTypeStr=boolean
  Compare To Constant2 : simulink/Logic and Bit Operations/Compare To Constant  relop===  const=0  OutDataTypeStr=boolean
  Compare To Constant3 : simulink/Logic and Bit Operations/Compare To Constant  relop=<  const=255  OutDataTypeStr=boolean
  Compare To Constant4 : simulink/Logic and Bit Operations/Compare To Constant  relop===  const=255  OutDataTypeStr=boolean
  Compare To Constant5 : simulink/Logic and Bit Operations/Compare To Constant  relop===  const=255  OutDataTypeStr=boolean
  Constant : Constant  OutDataTypeStr=uint8  SampleTime=-1
  Constant{1..4,12} (5 alike) : Constant  Value=0  OutDataTypeStr=uint8  SampleTime=-1
  Constant14 : Constant  OutDataTypeStr=uint8  SampleTime=-1
  Constant5 : Constant  Value=o1  OutDataTypeStr=uint8  SampleTime=-1
  Data Type Conversion : DataTypeConversion  OutDataTypeStr=boolean  SaturateOnIntegerOverflow=off  RndMeth=Floor
  Data Type Conversion4 : DataTypeConversion  OutDataTypeStr=fixdt(0,32,0)  SaturateOnIntegerOverflow=off  RndMeth=Floor
  Delay{1..3,5..6,8,18,40} (8 alike) : Delay  DelayLength=1
  Delay{4,7,10..12,19..22} (9 alike) : Delay
  Delay13 : Delay  DelayLength=3
  Delay{14..17} (4 alike) : Delay  DelayLength=44
  Delay9 : Delay  DelayLength=3
  HDL Counter1 : hdlsllib/Sources/HDL Counter  CountType=Free running  CountInit=0  CountStep=-1  CountMax=25  CountFromType=Initial value  CountFrom=0  CountResetPort=on  CountLoadPort=on  CountEnbPort=on  CountDirPort=off  CountHitOutputPort=off  CountDataType=Unsigned  CountWordLen=8  CountFracLen=0  CountSampTime=1
  HDL Counter2 : hdlsllib/Sources/HDL Counter  CountType=Count limited  CountInit=0  CountStep=1  CountMax=1  CountFromType=Initial value  CountFrom=0  CountResetPort=on  CountLoadPort=off  CountEnbPort=on  CountDirPort=off  CountHitOutputPort=off  CountDataType=Unsigned  CountWordLen=8  CountFracLen=0  CountSampTime=1
  HDL Counter3 : hdlsllib/Sources/HDL Counter  CountType=Free running  CountInit=0  CountStep=1  CountMax=2  CountFromType=Initial value  CountFrom=0  CountResetPort=on  CountLoadPort=off  CountEnbPort=on  CountDirPort=off  CountHitOutputPort=off  CountDataType=Unsigned  CountWordLen=8  CountFracLen=0  CountSampTime=1
  HDL Counter7 : hdlsllib/Sources/HDL Counter  CountType=Free running  CountInit=0  CountStep=1  CountMax=255  CountFromType=Initial value  CountFrom=0  CountResetPort=on  CountLoadPort=off  CountEnbPort=on  CountDirPort=off  CountHitOutputPort=off  CountDataType=Unsigned  CountWordLen=8  CountFracLen=0  CountSampTime=1
  HDL FIFO : hdlsllib/HDL RAMs/HDL FIFO  fifo_size=255  mode=Classic  ratio=1  push_msg=Warning  pop_msg=Warning  show_empty=off  show_full=off  show_num=off  LabelModeActiveChoice_Mode=Classic  rst_port=off
  NOT : Logic  Operator=NOT  IconShape=distinctive  AllPortsSameDT=off  OutDataTypeStr=boolean
  OR : Logic  Operator=OR  IconShape=distinctive  AllPortsSameDT=off  OutDataTypeStr=boolean
  Product : Product  OutDataTypeStr=uint8
  Product1 : Product  OutDataTypeStr=fixdt(0,32,15)
  Reciprocal : Product  Inputs=/  RndMeth=Zero  SaturateOnIntegerOverflow=on
  Relational Operator : RelationalOperator  Operator===  OutDataTypeStr=boolean  RndMeth=Simplest  InputSameDT=off
  Relational Operator1 : RelationalOperator  Operator===  OutDataTypeStr=boolean  RndMeth=Simplest  InputSameDT=off
  Relational Operator3 : RelationalOperator  Operator=<  OutDataTypeStr=boolean  RndMeth=Simplest  InputSameDT=off
  Simple Dual Port RAM : hdlsllib/HDL RAMs/Simple Dual Port RAM  ram_size=8
  Subtract : Sum  Inputs=+-
  Switch{,1,9,11} (4 alike) : Switch  Criteria=u2 ~= 0  SaturateOnIntegerOverflow=off  InputSameDT=off
  Switch12 : Switch  Criteria=u2 > Threshold  SaturateOnIntegerOverflow=off  InputSameDT=off
  t1 : Outport
  t1Enable : Outport  Port=2
  i1Val : Outport  Port=3
  wires:
  Delay6/1 -> Switch9/1
  Switch9/1 -> Delay8/1
  Switch1/1 -> Delay5/1
  Constant12/1 -> Switch9/3
  AND/1 -> NOT/1, HDL Counter1/1
  HDL Counter2/1 -> Data Type Conversion/1
  Compare To Constant2/1 -> AND/1
  enablei1/1 -> Simple Dual Port RAM/3, HDL Counter1/2, HDL Counter2/2
  Delay2/1 -> Subtract/2
  Subtract/1 -> Switch/3, Relational Operator/1, Delay1/1
  Reciprocal/1 -> Delay14/1
  Data Type Conversion4/1 -> Reciprocal/1
  Constant5/1 -> Product1/2
  Product1/1 -> Delay4/1
  Delay3/1 -> Product1/1
  Product/1 -> Delay19/1
  Delay5/1 -> Delay15/1
  Delay4/1 -> Product/2
  HDL Counter1/1 -> Compare To Constant2/1, Delay2/1
  i1/1 -> " Delay4"/1
  Data Type Conversion/1 -> AND1/1, HDL Counter3/2
  HDL Counter3/1 -> Compare To Constant4/1, Compare To Constant3/1, Compare To Constant1/1
  Compare To Constant1/1 -> HDL Counter2/1
  Compare To Constant3/1 -> AND1/2
  AND1/1 -> Delay12/1, HDL Counter1/4, AND/2
  " Delay3"/1 -> Switch1/1
  Constant1/1 -> Switch1/3
  Delay12/1 -> AND2/2
  AND2/1 -> Switch1/2, Delay16/1
  Constant2/1 -> Switch12/3
  i2HighEnable/1 -> HDL Counter7/2, Switch12/2, AND5/2
  Constant14/1 -> Add3/2
  Switch12/1 -> Relational Operator3/1
  Add3/1 -> Relational Operator3/2
  AND5/1 -> Delay10/1
  Relational Operator3/1 -> AND5/1
  Delay7/1 -> Switch9/2
  NOT/1 -> Delay13/1
  Delay13/1 -> AND2/1
  Delay10/1 -> Delay22/1
  HDL FIFO/1 -> Delay40/1
  Delay9/1 -> HDL FIFO/2
  Delay8/1 -> HDL FIFO/1
  Constant4/1 -> Switch11/3
  Delay40/1 -> Switch11/1
  Delay11/1 -> OR/2, Switch11/2
  OR/1 -> t1Enable/1
  Compare To Constant4/1 -> HDL Counter3/1
  HDL Counter7/1 -> Compare To Constant5/1, Switch12/1
  Compare To Constant5/1 -> HDL Counter7/1
  Constant/1 -> Delay18/1, Simple Dual Port RAM/2
  Delay18/1 -> Simple Dual Port RAM/4
  Switch/1 -> " Delay3"/1
  Relational Operator/1 -> AND3/1
  Delay1/1 -> Relational Operator1/2, Relational Operator/2
  Relational Operator1/1 -> AND3/2
  AND3/1 -> Switch/2
  Constant3/1 -> Switch/1
  " Delay4"/1 -> Simple Dual Port RAM/1, HDL Counter1/3
  Simple Dual Port RAM/1 -> Add3/1, Data Type Conversion4/1, i1Val/1, Relational Operator1/1, Subtract/1
  Delay14/1 -> Delay3/1
  Delay16/1 -> Delay21/1, Delay20/1
  Delay17/1 -> Delay11/1, HDL FIFO/3
  Delay19/1 -> Delay6/1
  Delay20/1 -> Delay7/1
  Delay21/1 -> Delay9/1
  Delay22/1 -> Delay17/1
  Switch11/1 -> t1/1, OR/1
  Delay15/1 -> Product/1

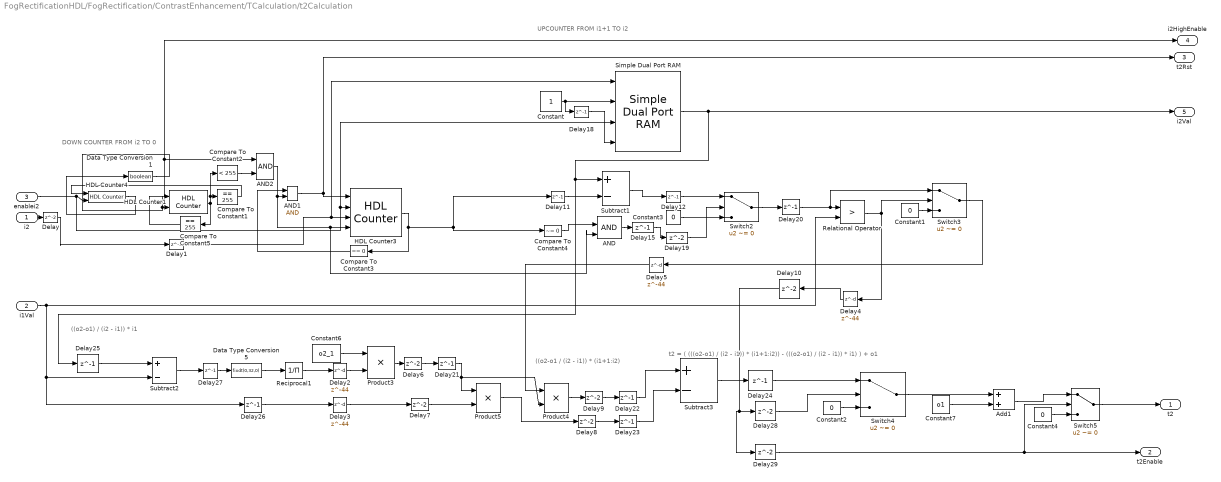
== system FogRectificationHDL/FogRectification/ContrastEnhancement/TCalculation/t2Calculation ==
  note: ((o2-o1) / (i2 - i1)) * i1
  note: UPCOUNTER FROM i1+1 TO i2
  note: DOWN COUNTER FROM i2 TO 0
  note: ((o2-o1 / (i2 - i1)) * (i1+1:i2)
  note: t2 = ( (((o2-o1) / (i2 - i1)) * (i1+1:i2)) - (((o2-o1) / (i2 - i1)) * i1) ) + o1
  i2 : Inport
  i1Val : Inport  Port=2
  enablei2 : Inport  Port=3
  AND : Logic  IconShape=distinctive  AllPortsSameDT=off  OutDataTypeStr=boolean
  AND1 : Logic  IconShape=distinctive  AllPortsSameDT=off  OutDataTypeStr=boolean
  AND2 : Logic  IconShape=distinctive  AllPortsSameDT=off  OutDataTypeStr=boolean
  Add1 : Sum  OutDataTypeStr=uint8
  Compare To Constant1 : simulink/Logic and Bit Operations/Compare To Constant  relop===  const=255  OutDataTypeStr=boolean
  Compare To Constant2 : simulink/Logic and Bit Operations/Compare To Constant  relop=<  const=255  OutDataTypeStr=boolean
  Compare To Constant3 : simulink/Logic and Bit Operations/Compare To Constant  relop===  const=0  OutDataTypeStr=boolean
  Compare To Constant4 : simulink/Logic and Bit Operations/Compare To Constant  relop=~=  const=0  OutDataTypeStr=boolean
  Compare To Constant5 : simulink/Logic and Bit Operations/Compare To Constant  relop===  const=255  OutDataTypeStr=boolean
  Constant : Constant  OutDataTypeStr=uint8  SampleTime=-1
  Constant{1..4} (4 alike) : Constant  Value=0  OutDataTypeStr=uint8  SampleTime=-1
  Constant6 : Constant  Value=o2_1  OutDataTypeStr=uint8  SampleTime=-1
  Constant7 : Constant  Value=o1  OutDataTypeStr=uint8  SampleTime=-1
  Data Type Conversion1 : DataTypeConversion  OutDataTypeStr=boolean  SaturateOnIntegerOverflow=off  RndMeth=Floor
  Data Type Conversion5 : DataTypeConversion  OutDataTypeStr=fixdt(0,32,0)  SaturateOnIntegerOverflow=off  RndMeth=Floor
  Delay{,6..10,19,28..29} (9 alike) : Delay
  Delay{1,11..12,15,18,20..27} (13 alike) : Delay  DelayLength=1
  Delay{2..5} (4 alike) : Delay  DelayLength=44
  HDL Counter1 : hdlsllib/Sources/HDL Counter  CountType=Free running  CountInit=0  CountStep=1  CountMax=1  CountFromType=Initial value  CountFrom=0  CountResetPort=on  CountLoadPort=off  CountEnbPort=on  CountDirPort=off  CountHitOutputPort=off  CountDataType=Unsigned  CountWordLen=8  CountFracLen=0  CountSampTime=1
  HDL Counter3 : hdlsllib/Sources/HDL Counter  CountType=Free running  CountInit=0  CountStep=-1  CountMax=25  CountFromType=Initial value  CountFrom=0  CountResetPort=on  CountLoadPort=on  CountEnbPort=on  CountDirPort=off  CountHitOutputPort=off  CountDataType=Unsigned  CountWordLen=8  CountFracLen=0  CountSampTime=1
  HDL Counter4 : hdlsllib/Sources/HDL Counter  CountType=Count limited  CountInit=0  CountStep=1  CountMax=1  CountFromType=Initial value  CountFrom=0  CountResetPort=on  CountLoadPort=off  CountEnbPort=on  CountDirPort=off  CountHitOutputPort=off  CountDataType=Unsigned  CountWordLen=8  CountFracLen=0  CountSampTime=1
  Product3 : Product  OutDataTypeStr=fixdt(0,32,15)
  Product4 : Product  OutDataTypeStr=fixdt(0,32,15)
  Product5 : Product  OutDataTypeStr=fixdt(0,32,15)
  Reciprocal1 : Product  Inputs=/  RndMeth=Zero  SaturateOnIntegerOverflow=on
  Relational Operator : RelationalOperator  Operator=>  OutDataTypeStr=boolean  RndMeth=Simplest  InputSameDT=off
  Simple Dual Port RAM : hdlsllib/HDL RAMs/Simple Dual Port RAM  ram_size=8
  Subtract1 : Sum  Inputs=+-  AccumDataTypeStr=uint8
  Subtract2 : Sum  Inputs=+-
  Subtract3 : Sum  Inputs=+-
  Switch{2..5} (4 alike) : Switch  Criteria=u2 ~= 0  SaturateOnIntegerOverflow=off  InputSameDT=off
  t2 : Outport
  t2Enable : Outport  Port=2
  t2Rst : Outport  Port=3
  i2HighEnable : Outport  Port=4
  i2Val : Outport  Port=5
  wires:
  Constant7/1 -> Add1/2
  Switch4/1 -> Add1/1
  Product5/1 -> Delay8/1
  Constant4/1 -> Switch5/3
  Add1/1 -> Switch5/1
  Delay22/1 -> Subtract3/1
  Delay26/1 -> Delay3/1
  Delay28/1 -> Switch4/2
  Delay23/1 -> Subtract3/2
  Delay24/1 -> Switch4/1
  Subtract3/1 -> Delay24/1
  Switch5/1 -> t2/1
  Compare To Constant3/1 -> AND1/1
  enablei2/1 -> HDL Counter4/2, HDL Counter3/2, Simple Dual Port RAM/3
  HDL Counter4/1 -> Data Type Conversion1/1
  Relational Operator/1 -> Switch3/2, Delay4/1
  HDL Counter3/1 -> Compare To Constant4/1, Delay11/1, Compare To Constant3/1
  Subtract1/1 -> Delay12/1
  Simple Dual Port RAM/1 -> i2Val/1, Delay25/1, Subtract1/1
  Delay19/1 -> Switch2/2
  Constant1/1 -> Switch3/3
  Delay15/1 -> Delay19/1
  Delay20/1 -> Relational Operator/1, Switch3/1
  Switch2/1 -> Delay20/1
  Delay11/1 -> Subtract1/2
  Constant6/1 -> Product3/1
  Delay27/1 -> Data Type Conversion5/1
  Data Type Conversion5/1 -> Reciprocal1/1
  Delay25/1 -> Subtract2/1
  Reciprocal1/1 -> Delay2/1
  i1Val/1 -> Delay26/1, Subtract2/2, Relational Operator/2
  Subtract2/1 -> Delay27/1
  Delay21/1 -> Product4/2, Product5/1
  Product4/1 -> Delay9/1
  Constant2/1 -> Switch4/3
  AND1/1 -> HDL Counter3/1, t2Rst/1
  Data Type Conversion1/1 -> AND2/1, i2HighEnable/1, HDL Counter1/2
  HDL Counter1/1 -> Compare To Constant5/1, Compare To Constant2/1, Compare To Constant1/1
  Compare To Constant1/1 -> HDL Counter4/1
  Compare To Constant2/1 -> AND2/2
  AND2/1 -> AND/2, HDL Counter3/4, AND1/2
  Delay12/1 -> Switch2/1
  Constant3/1 -> Switch2/3
  Compare To Constant4/1 -> AND/1
  AND/1 -> Delay15/1
  Switch3/1 -> Delay5/1
  i2/1 -> Delay/1
  Delay/1 -> Delay1/1
  Compare To Constant5/1 -> HDL Counter1/1
  Constant/1 -> Simple Dual Port RAM/2, Delay18/1
  Delay18/1 -> Simple Dual Port RAM/4
  Delay1/1 -> Simple Dual Port RAM/1, HDL Counter3/3
  Delay2/1 -> Product3/2
  Delay3/1 -> Delay7/1
  Delay4/1 -> Delay10/1
  Delay5/1 -> Product4/1
  Product3/1 -> Delay6/1
  Delay6/1 -> Delay21/1
  Delay7/1 -> Product5/2
  Delay8/1 -> Delay23/1
  Delay9/1 -> Delay22/1
  Delay10/1 -> Delay29/1, Delay28/1
  Delay29/1 -> Switch5/2, t2Enable/1

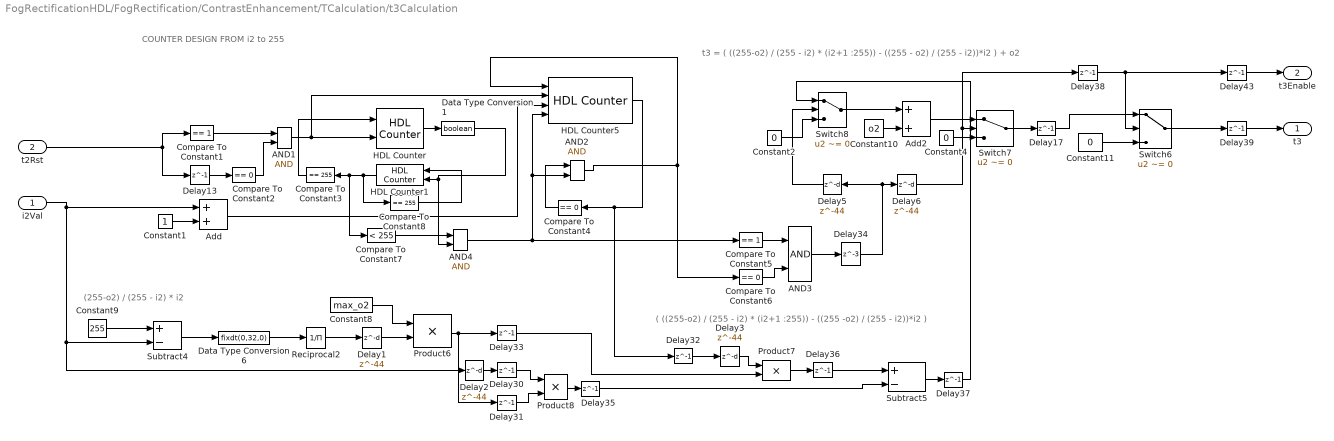
== system FogRectificationHDL/FogRectification/ContrastEnhancement/TCalculation/t3Calculation ==
  note: COUNTER DESIGN FROM i2 to 255
  note: (255-o2) / (255 - i2) * i2
  note: ( ((255-o2) / (255 - i2) * (i2+1 :255)) - ((255 -o2) / (255 - i2))*i2 )
  note: t3 = ( ((255-o2) / (255 - i2) * (i2+1 :255)) - ((255 - o2) / (255 - i2))*i2 ) + o2
  i2Val : Inport
  t2Rst : Inport  Port=2
  AND{1..4} (4 alike) : Logic  IconShape=distinctive  AllPortsSameDT=off  OutDataTypeStr=boolean
  Add : Sum  OutDataTypeStr=uint8
  Add2 : Sum  OutDataTypeStr=uint8
  Compare To Constant1 : simulink/Logic and Bit Operations/Compare To Constant  relop===  const=1  OutDataTypeStr=boolean
  Compare To Constant2 : simulink/Logic and Bit Operations/Compare To Constant  relop===  const=0  OutDataTypeStr=boolean
  Compare To Constant3 : simulink/Logic and Bit Operations/Compare To Constant  relop===  const=255  OutDataTypeStr=boolean
  Compare To Constant4 : simulink/Logic and Bit Operations/Compare To Constant  relop===  const=0  OutDataTypeStr=boolean
  Compare To Constant5 : simulink/Logic and Bit Operations/Compare To Constant  relop===  const=1  OutDataTypeStr=boolean
  Compare To Constant6 : simulink/Logic and Bit Operations/Compare To Constant  relop===  const=0  OutDataTypeStr=boolean
  Compare To Constant7 : simulink/Logic and Bit Operations/Compare To Constant  relop=<  const=255  OutDataTypeStr=boolean
  Compare To Constant8 : simulink/Logic and Bit Operations/Compare To Constant  relop===  const=255  OutDataTypeStr=boolean
  Constant1 : Constant  OutDataTypeStr=uint8  SampleTime=-1
  Constant10 : Constant  Value=o2  OutDataTypeStr=uint8  SampleTime=-1
  Constant11 : Constant  Value=0  OutDataTypeStr=uint8  SampleTime=-1
  Constant2 : Constant  Value=0  OutDataTypeStr=uint8  SampleTime=-1
  Constant4 : Constant  Value=0  OutDataTypeStr=uint8  SampleTime=-1
  Constant8 : Constant  Value=max_o2  OutDataTypeStr=uint8  SampleTime=-1
  Constant9 : Constant  Value=255  OutDataTypeStr=uint8  SampleTime=-1
  Data Type Conversion1 : DataTypeConversion  OutDataTypeStr=boolean  SaturateOnIntegerOverflow=off  RndMeth=Floor
  Data Type Conversion6 : DataTypeConversion  OutDataTypeStr=fixdt(0,32,0)  SaturateOnIntegerOverflow=off  RndMeth=Floor
  Delay{1..3,5..6} (5 alike) : Delay  DelayLength=44
  Delay{13,17,30..33,35..39,43} (12 alike) : Delay  DelayLength=1
  Delay34 : Delay  DelayLength=3
  HDL Counter : hdlsllib/Sources/HDL Counter  CountType=Count limited  CountInit=0  CountStep=1  CountMax=1  CountFromType=Initial value  CountFrom=0  CountResetPort=on  CountLoadPort=off  CountEnbPort=on  CountDirPort=off  CountHitOutputPort=off  CountDataType=Unsigned  CountWordLen=8  CountFracLen=0  CountSampTime=1
  HDL Counter1 : hdlsllib/Sources/HDL Counter  CountType=Free running  CountInit=0  CountStep=1  CountMax=1  CountFromType=Initial value  CountFrom=0  CountResetPort=on  CountLoadPort=off  CountEnbPort=on  CountDirPort=off  CountHitOutputPort=off  CountDataType=Unsigned  CountWordLen=8  CountFracLen=0  CountSampTime=1
  HDL Counter5 : hdlsllib/Sources/HDL Counter  CountType=Free running  CountInit=0  CountStep=1  CountMax=25  CountFromType=Initial value  CountFrom=0  CountResetPort=on  CountLoadPort=on  CountEnbPort=on  CountDirPort=off  CountHitOutputPort=off  CountDataType=Unsigned  CountWordLen=8  CountFracLen=0  CountSampTime=1
  Product6 : Product  OutDataTypeStr=fixdt(0,32,15)
  Product7 : Product  OutDataTypeStr=fixdt(0,32,15)
  Product8 : Product  OutDataTypeStr=fixdt(0,32,15)
  Reciprocal2 : Product  Inputs=/  RndMeth=Zero  SaturateOnIntegerOverflow=on
  Subtract4 : Sum  Inputs=+-
  Subtract5 : Sum  Inputs=+-
  Switch6 : Switch  Criteria=u2 ~= 0  SaturateOnIntegerOverflow=off  InputSameDT=off
  Switch7 : Switch  Criteria=u2 ~= 0  SaturateOnIntegerOverflow=off  InputSameDT=off
  Switch8 : Switch  Criteria=u2 ~= 0  SaturateOnIntegerOverflow=off  InputSameDT=off
  t3 : Outport
  t3Enable : Outport  Port=2
  wires:
  Constant10/1 -> Add2/2
  Delay32/1 -> Delay3/1
  Delay38/1 -> Switch6/2, Delay43/1
  Product6/1 -> Delay33/1, Delay31/1
  Delay39/1 -> t3/1
  Product8/1 -> Delay35/1
  Product7/1 -> Delay36/1
  Delay35/1 -> Subtract5/2
  Delay36/1 -> Subtract5/1
  Delay30/1 -> Product8/1
  Delay33/1 -> Product7/2
  Constant8/1 -> Product6/1
  Constant11/1 -> Switch6/3
  Subtract5/1 -> Delay37/1
  Data Type Conversion6/1 -> Reciprocal2/1
  Switch6/1 -> Delay39/1
  Delay37/1 -> Switch8/1
  AND3/1 -> Delay34/1
  Delay17/1 -> Switch6/1
  Constant9/1 -> Subtract4/1
  Switch8/1 -> Add2/1
  Subtract4/1 -> Data Type Conversion6/1
  Add2/1 -> Switch7/1
  Switch7/1 -> Delay17/1
  Delay31/1 -> Product8/2
  Delay43/1 -> t3Enable/1
  Constant2/1 -> Switch8/3
  Constant4/1 -> Switch7/3
  Compare To Constant5/1 -> AND3/1
  Compare To Constant6/1 -> AND3/2
  AND4/1 -> HDL Counter5/4, AND2/2, Compare To Constant5/1
  AND2/1 -> Compare To Constant6/1, HDL Counter5/1
  Delay13/1 -> Compare To Constant2/1
  Compare To Constant7/1 -> AND4/1
  Compare To Constant1/1 -> AND1/1
  HDL Counter/1 -> Data Type Conversion1/1
  Data Type Conversion1/1 -> AND4/2, HDL Counter1/2
  Compare To Constant4/1 -> AND2/1
  Constant1/1 -> Add/2
  Add/1 -> HDL Counter5/3
  AND1/1 -> HDL Counter/2, HDL Counter5/2
  Compare To Constant2/1 -> AND1/2
  Compare To Constant3/1 -> HDL Counter/1
  HDL Counter1/1 -> Compare To Constant8/1, Compare To Constant7/1, Compare To Constant3/1
  t2Rst/1 -> Compare To Constant1/1, Delay13/1
  Compare To Constant8/1 -> HDL Counter1/1
  Reciprocal2/1 -> Delay1/1
  i2Val/1 -> Delay2/1, Subtract4/2, Add/1
  HDL Counter5/1 -> Delay32/1, Compare To Constant4/1
  Delay34/1 -> Delay5/1, Delay6/1
  Delay1/1 -> Product6/2
  Delay2/1 -> Delay30/1
  Delay3/1 -> Product7/1
  Delay5/1 -> Switch8/2
  Delay6/1 -> Delay38/1, Switch7/2
